simulink library "posemodel"  (R2019b)
settings: Solver=VariableStepAuto  StartTime=0.0  StopTime=10.0  RelTol=1e-3
libraries: posefilter x14, timecompensate x1

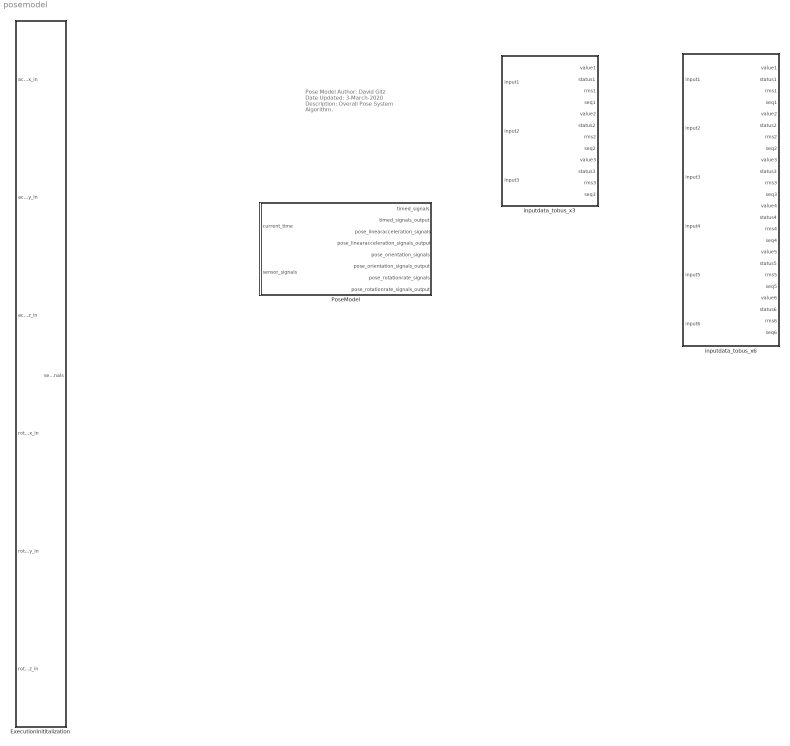
== system posemodel ==
  note: Pose Model
      | Author: David Gitz
      | Date Updated: 3-March-2020
      | Description:
      | Overall Pose System Algorithm.
  ExecutionInititalization : Subsystem
  PoseModel : Subsystem
  inputdata_tobus_x3 : MATLAB Function  TreatAsAtomicUnit=on
  inputdata_tobus_x6 : MATLAB Function  TreatAsAtomicUnit=on

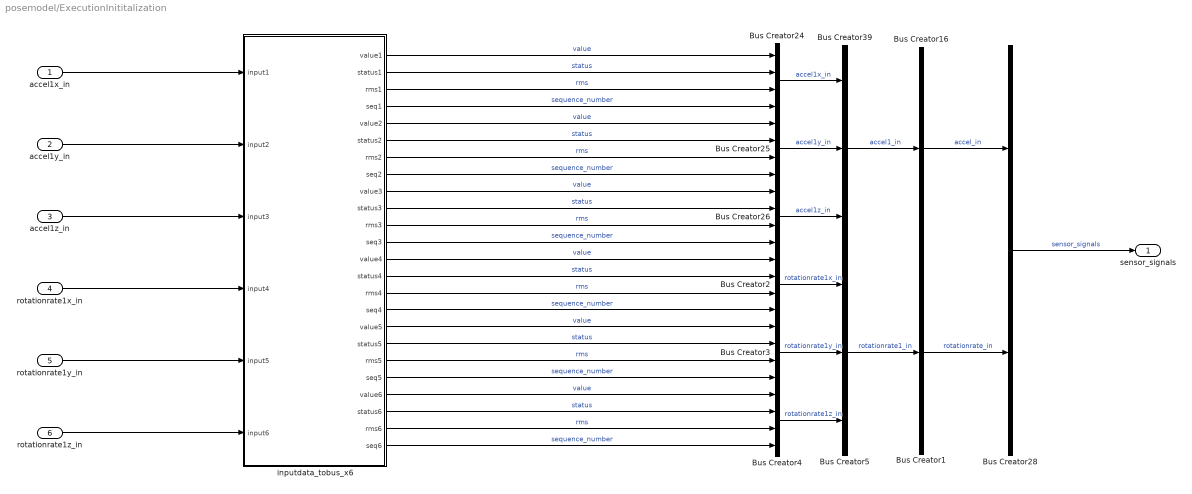
== system posemodel/ExecutionInititalization ==
  accel1x_in : Inport
  accel1y_in : Inport  Port=2
  accel1z_in : Inport  Port=3
  rotationrate1x_in : Inport  Port=4
  rotationrate1y_in : Inport  Port=5
  rotationrate1z_in : Inport  Port=6
  Bus Creator1 : BusCreator  Inputs=1
  Bus Creator16 : BusCreator  Inputs=1
  Bus Creator{2..4,24..26} (6 alike) : BusCreator  Inputs=4  OutDataTypeStr=Bus: InputSignalObject
  Bus Creator28 : BusCreator  Inputs=2
  Bus Creator39 : BusCreator  Inputs=3
  Bus Creator5 : BusCreator  Inputs=3
  inputdata_tobus_x6 : MATLAB Function  TreatAsAtomicUnit=on
  sensor_signals : Outport
  wires:
  inputdata_tobus_x6/20(seq5) -> Bus Creator3/4  "sequence_number"
  inputdata_tobus_x6/22(status6) -> Bus Creator4/2  "status"
  inputdata_tobus_x6/13(value4) -> Bus Creator2/1  "value"
  Bus Creator4/1 -> Bus Creator5/3  "rotationrate1z_in"
  Bus Creator1/1 -> Bus Creator28/2  "rotationrate_in"
  Bus Creator2/1 -> Bus Creator5/1  "rotationrate1x_in"
  inputdata_tobus_x6/23(rms6) -> Bus Creator4/3  "rms"
  inputdata_tobus_x6/14(status4) -> Bus Creator2/2  "status"
  inputdata_tobus_x6/21(value6) -> Bus Creator4/1  "value"
  inputdata_tobus_x6/19(rms5) -> Bus Creator3/3  "rms"
  inputdata_tobus_x6/17(value5) -> Bus Creator3/1  "value"
  Bus Creator5/1 -> Bus Creator1/1  "rotationrate1_in"
  inputdata_tobus_x6/16(seq4) -> Bus Creator2/4  "sequence_number"
  inputdata_tobus_x6/24(seq6) -> Bus Creator4/4  "sequence_number"
  inputdata_tobus_x6/15(rms4) -> Bus Creator2/3  "rms"
  inputdata_tobus_x6/18(status5) -> Bus Creator3/2  "status"
  Bus Creator3/1 -> Bus Creator5/2  "rotationrate1y_in"
  rotationrate1y_in/1 -> inputdata_tobus_x6/5(input5)
  rotationrate1z_in/1 -> inputdata_tobus_x6/6(input6)
  rotationrate1x_in/1 -> inputdata_tobus_x6/4(input4)
  inputdata_tobus_x6/3(rms1) -> Bus Creator24/3  "rms"
  inputdata_tobus_x6/5(value2) -> Bus Creator25/1  "value"
  inputdata_tobus_x6/2(status1) -> Bus Creator24/2  "status"
  inputdata_tobus_x6/4(seq1) -> Bus Creator24/4  "sequence_number"
  inputdata_tobus_x6/11(rms3) -> Bus Creator26/3  "rms"
  inputdata_tobus_x6/12(seq3) -> Bus Creator26/4  "sequence_number"
  Bus Creator39/1 -> Bus Creator16/1  "accel1_in"
  Bus Creator28/1 -> sensor_signals/1  "sensor_signals"
  accel1x_in/1 -> inputdata_tobus_x6/1(input1)
  inputdata_tobus_x6/6(status2) -> Bus Creator25/2  "status"
  accel1z_in/1 -> inputdata_tobus_x6/3(input3)
  Bus Creator24/1 -> Bus Creator39/1  "accel1x_in"
  Bus Creator16/1 -> Bus Creator28/1  "accel_in"
  Bus Creator25/1 -> Bus Creator39/2  "accel1y_in"
  inputdata_tobus_x6/9(value3) -> Bus Creator26/1  "value"
  inputdata_tobus_x6/7(rms2) -> Bus Creator25/3  "rms"
  inputdata_tobus_x6/8(seq2) -> Bus Creator25/4  "sequence_number"
  Bus Creator26/1 -> Bus Creator39/3  "accel1z_in"
  accel1y_in/1 -> inputdata_tobus_x6/2(input2)
  inputdata_tobus_x6/1(value1) -> Bus Creator24/1  "value"
  inputdata_tobus_x6/10(status3) -> Bus Creator26/2  "status"

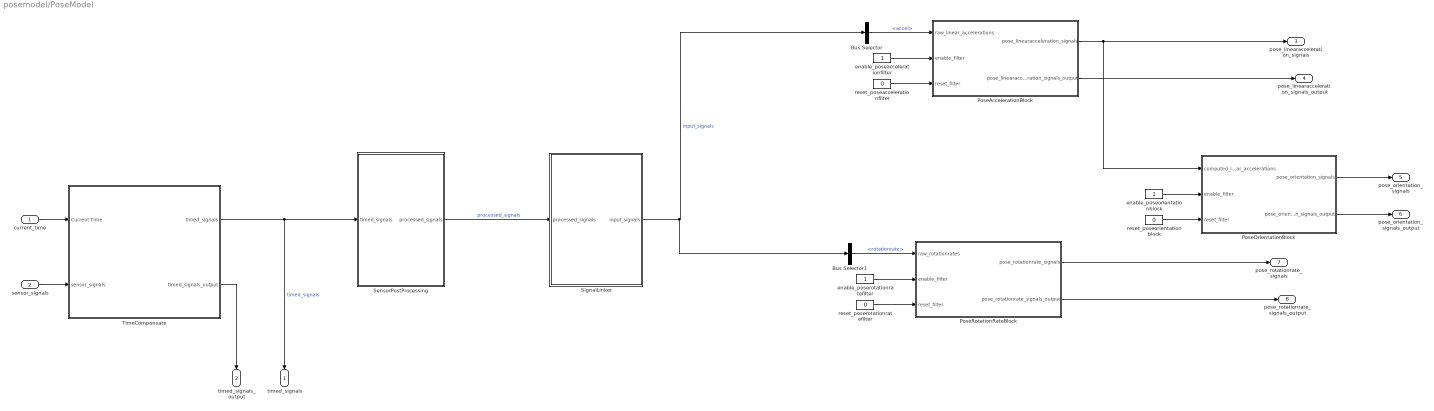
== system posemodel/PoseModel ==
  current_time : Inport
  sensor_signals : Inport  Port=2
  Bus Selector : BusSelector  OutputSignals=accel
  Bus Selector1 : BusSelector  OutputSignals=rotationrate
  PoseAccelerationBlock : Subsystem
  PoseOrientationBlock : Subsystem
  PoseRotationRateBlock : Subsystem
  SensorPostProcessing : Subsystem
  SignalLinker : Subsystem
  TimeCompensate : Subsystem  TreatAsAtomicUnit=on
  enable_poseaccelerationfilter : Constant
  enable_poseorientationblock : Constant
  enable_poserotationratefilter : Constant
  reset_poseaccelerationfilter : Constant  Value=0
  reset_poseorientationblock : Constant  Value=0
  reset_poserotationratefilter : Constant  Value=0
  timed_signals : Outport
  timed_signals_output : Outport  Port=2
  pose_linearacceleration_signals : Outport  Port=3
  pose_linearacceleration_signals_output : Outport  Port=4
  pose_orientation_signals : Outport  Port=5
  pose_orientation_signals_output : Outport  Port=6
  pose_rotationrate_signals : Outport  Port=7
  pose_rotationrate_signals_output : Outport  Port=8
  wires:
  PoseRotationRateBlock/1(pose_rotationrate_signals) -> pose_rotationrate_signals/1
  Bus Selector1/1 -> PoseRotationRateBlock/1(raw_rotationrates)  "<rotationrate>"
  enable_poserotationratefilter/1 -> PoseRotationRateBlock/2(enable_filter)
  reset_poserotationratefilter/1 -> PoseRotationRateBlock/3(reset_filter)
  PoseRotationRateBlock/2(pose_rotationrate_signals_output) -> pose_rotationrate_signals_output/1
  PoseAccelerationBlock/2(pose_linearacceleration_signals_output) -> pose_linearacceleration_signals_output/1
  TimeCompensate/2(timed_signals_output) -> timed_signals_output/1
  PoseOrientationBlock/2(pose_orientation_signals_output) -> pose_orientation_signals_output/1
  PoseOrientationBlock/1(pose_orientation_signals) -> pose_orientation_signals/1
  reset_poseorientationblock/1 -> PoseOrientationBlock/3(reset_filter)
  enable_poseorientationblock/1 -> PoseOrientationBlock/2(enable_filter)
  reset_poseaccelerationfilter/1 -> PoseAccelerationBlock/3(reset_filter)
  enable_poseaccelerationfilter/1 -> PoseAccelerationBlock/2(enable_filter)
  current_time/1 -> TimeCompensate/1(Current Time)
  Bus Selector/1 -> PoseAccelerationBlock/1(raw_linear_accelerations)  "<accel>"
  PoseAccelerationBlock/1(pose_linearacceleration_signals) -> pose_linearacceleration_signals/1, PoseOrientationBlock/1(computed_linear_accelerations)
  sensor_signals/1 -> TimeCompensate/2(sensor_signals)
  SensorPostProcessing/1(processed_signals) -> SignalLinker/1(processed_signals)  "processed_signals"
  SignalLinker/1(input_signals) -> Bus Selector/1, Bus Selector1/1  "input_signals"
  TimeCompensate/1(timed_signals) -> timed_signals/1, SensorPostProcessing/1(timed_signals)  "timed_signals"

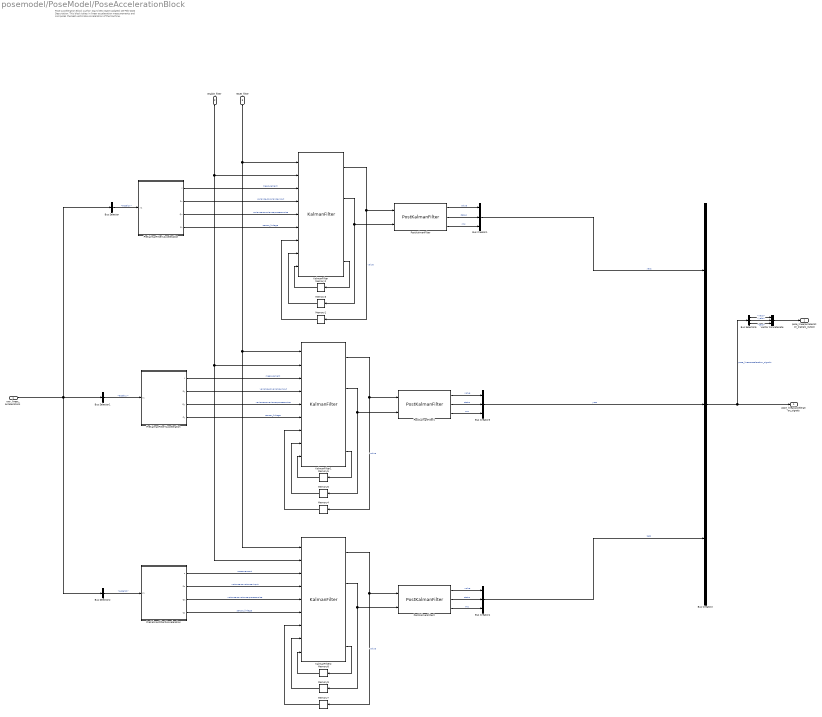
== system posemodel/PoseModel/PoseAccelerationBlock ==
  note: Pose Acceleration Block
      | Author: David Gitz
      | Date Updated: 28-Feb-2020
      | Description:
      | This block takes in linear acceleration measurements and computes the
      | best-estimate Acceleration of the Machine.
  raw_linear_accelerations : Inport
  enable_filter : Inport  Port=2
  reset_filter : Inport  Port=3
  Bus Creator1 : BusCreator  Inputs=3  OutDataTypeStr=Bus: OutputSignalObject  NonVirtualBus=on
  Bus Creator2 : BusCreator  Inputs=3
  Bus Creator3 : BusCreator  Inputs=3  OutDataTypeStr=Bus: OutputSignalObject  NonVirtualBus=on
  Bus Creator4 : BusCreator  Inputs=3  OutDataTypeStr=Bus: OutputSignalObject  NonVirtualBus=on
  Bus Selector : BusSelector  OutputSignals=accel1.accel1x
  Bus Selector1 : BusSelector  OutputSignals=accel1.accel1y
  Bus Selector2 : BusSelector  OutputSignals=accel1.accel1z
  Bus Selector6 : BusSelector  OutputSignals=xacc,yacc,zacc
  KalmanFilter : posefilter/KalmanFilter  SystemSampleTime=-1  Latency=0  AutoFrameSizeCalculation=off
  KalmanFilter1 : posefilter/KalmanFilter  SystemSampleTime=-1  Latency=0  AutoFrameSizeCalculation=off
  KalmanFilter2 : posefilter/KalmanFilter  SystemSampleTime=-1  Latency=0  AutoFrameSizeCalculation=off
  Memory{1..9} (9 alike) : Memory
  PostKalmanFilter : posefilter/PostKalmanFilter  SystemSampleTime=-1  Latency=0  AutoFrameSizeCalculation=off
  PostKalmanFilter1 : posefilter/PostKalmanFilter  SystemSampleTime=-1  Latency=0  AutoFrameSizeCalculation=off
  PostKalmanFilter2 : posefilter/PostKalmanFilter  SystemSampleTime=-1  Latency=0  AutoFrameSizeCalculation=off
  PreKalmanFilterXAcceleration : MATLAB Function  TreatAsAtomicUnit=on
  PreKalmanFilterYAcceleration : MATLAB Function  TreatAsAtomicUnit=on
  PreKalmanFilterZAcceleration : MATLAB Function  TreatAsAtomicUnit=on
  Vector Concatenate : Concatenate  NumInputs=3
  pose_linearacceleration_signals : Outport
  pose_linearacceleration_signals_output : Outport  Port=2
  wires:
  Vector Concatenate/1 -> pose_linearacceleration_signals_output/1
  Bus Selector6/3 -> Vector Concatenate/3  "<zacc>"
  Bus Selector6/2 -> Vector Concatenate/2  "<yacc>"
  Bus Selector6/1 -> Vector Concatenate/1  "<xacc>"
  Bus Creator2/1 -> pose_linearacceleration_signals/1, Bus Selector6/1  "pose_linearacceleration_signals"
  PostKalmanFilter2/3 -> Bus Creator4/3  "rms"
  Memory9/1 -> KalmanFilter2/8
  KalmanFilter2/1 -> PostKalmanFilter2/1, Memory7/1  "value"
  PreKalmanFilterZAcceleration/1(z) -> KalmanFilter2/3  "measurement"
  PostKalmanFilter2/1 -> Bus Creator4/1  "value"
  PreKalmanFilterZAcceleration/2(Rz) -> KalmanFilter2/4  "variance-covariance-input"
  PostKalmanFilter2/2 -> Bus Creator4/2  "status"
  raw_linear_accelerations/1 -> Bus Selector1/1, Bus Selector/1, Bus Selector2/1
  reset_filter/1 -> KalmanFilter/1, KalmanFilter1/1, KalmanFilter2/1
  Bus Selector2/1 -> PreKalmanFilterZAcceleration/1(x1)  "<accel1z>"
  KalmanFilter2/4 -> Memory8/1
  KalmanFilter2/2 -> Memory9/1, PostKalmanFilter2/2
  Bus Creator4/1 -> Bus Creator2/3  "zacc"
  enable_filter/1 -> KalmanFilter/2, KalmanFilter1/2, KalmanFilter2/2
  PreKalmanFilterZAcceleration/3(Qz) -> KalmanFilter2/5  "variance-covariance-processnoise"
  Memory8/1 -> KalmanFilter2/9
  Memory7/1 -> KalmanFilter2/7
  PreKalmanFilterZAcceleration/4(Cz) -> KalmanFilter2/6  "sensor_linkage"
  Bus Creator3/1 -> Bus Creator2/2  "yacc"
  PreKalmanFilterYAcceleration/1(y) -> KalmanFilter1/3  "measurement"
  PostKalmanFilter1/3 -> Bus Creator3/3  "rms"
  Memory6/1 -> KalmanFilter1/8
  PostKalmanFilter1/2 -> Bus Creator3/2  "status"
  PostKalmanFilter1/1 -> Bus Creator3/1  "value"
  PreKalmanFilterYAcceleration/2(Ry) -> KalmanFilter1/4  "variance-covariance-input"
  Memory4/1 -> KalmanFilter1/7
  PreKalmanFilterYAcceleration/3(Qy) -> KalmanFilter1/5  "variance-covariance-processnoise"
  PreKalmanFilterYAcceleration/4(Cy) -> KalmanFilter1/6  "sensor_linkage"
  Bus Selector1/1 -> PreKalmanFilterYAcceleration/1(x1)  "<accel1y>"
  KalmanFilter1/1 -> PostKalmanFilter1/1, Memory4/1  "value"
  KalmanFilter1/2 -> Memory6/1, PostKalmanFilter1/2
  KalmanFilter1/4 -> Memory5/1
  Memory5/1 -> KalmanFilter1/9
  PreKalmanFilterXAcceleration/3(Qx) -> KalmanFilter/5  "variance-covariance-processnoise"
  PreKalmanFilterXAcceleration/1(x) -> KalmanFilter/3  "measurement"
  PreKalmanFilterXAcceleration/4(Cx) -> KalmanFilter/6  "sensor_linkage"
  KalmanFilter/2 -> Memory3/1, PostKalmanFilter/2
  Memory3/1 -> KalmanFilter/8
  Bus Selector/1 -> PreKalmanFilterXAcceleration/1(x1)  "<accel1x>"
  PostKalmanFilter/2 -> Bus Creator1/2  "status"
  PostKalmanFilter/1 -> Bus Creator1/1  "value"
  PostKalmanFilter/3 -> Bus Creator1/3  "rms"
  Memory2/1 -> KalmanFilter/9
  Memory1/1 -> KalmanFilter/7
  PreKalmanFilterXAcceleration/2(Rx) -> KalmanFilter/4  "variance-covariance-input"
  KalmanFilter/4 -> Memory2/1
  Bus Creator1/1 -> Bus Creator2/1  "xacc"
  KalmanFilter/1 -> PostKalmanFilter/1, Memory1/1  "value"

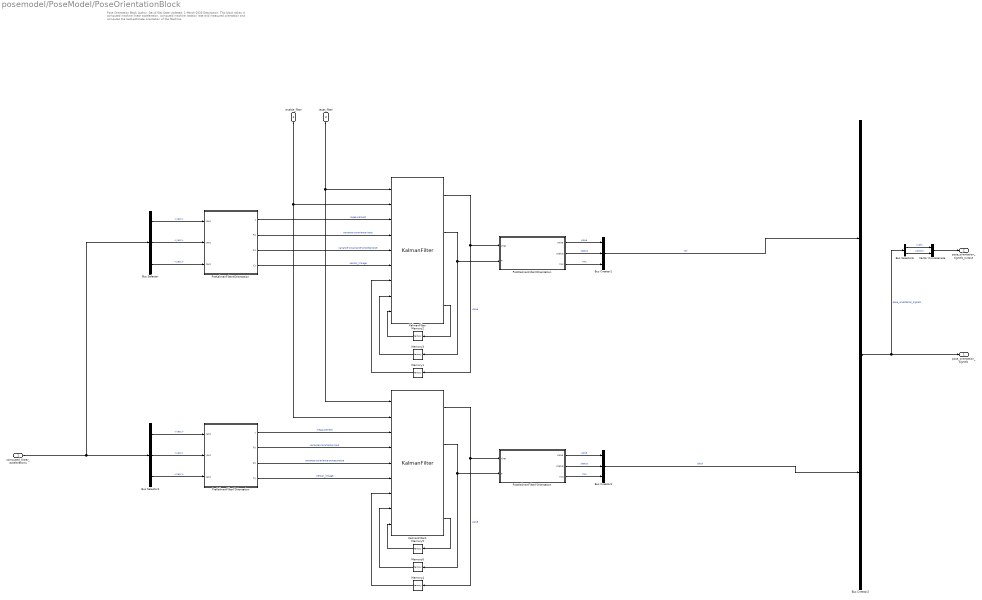
== system posemodel/PoseModel/PoseOrientationBlock ==
  note: Pose Orientation Block
      | Author: David Gitz
      | Date Updated: 1-March-2020
      | Description:
      | This block takes in computed machine linear acceleration, computed machine rotation rate and measured orientation and computes the
      | best-estimate orientation of the Machine.
  computed_linear_accelerations : Inport
  enable_filter : Inport  Port=2
  reset_filter : Inport  Port=3
  Bus Creator1 : BusCreator  Inputs=3  OutDataTypeStr=Bus: OutputSignalObject  NonVirtualBus=on
  Bus Creator2 : BusCreator  Inputs=2
  Bus Creator3 : BusCreator  Inputs=3  OutDataTypeStr=Bus: OutputSignalObject  NonVirtualBus=on
  Bus Selector : BusSelector  OutputSignals=xacc,yacc,zacc
  Bus Selector1 : BusSelector  OutputSignals=xacc,yacc,zacc
  Bus Selector6 : BusSelector  OutputSignals=roll,pitch
  KalmanFilter : posefilter/KalmanFilter  SystemSampleTime=-1  Latency=0  AutoFrameSizeCalculation=off
  KalmanFilter1 : posefilter/KalmanFilter  SystemSampleTime=-1  Latency=0  AutoFrameSizeCalculation=off
  Memory{1..6} (6 alike) : Memory
  PostKalmanFilterXOrientation : MATLAB Function  TreatAsAtomicUnit=on
  PostKalmanFilterYOrientation : MATLAB Function  TreatAsAtomicUnit=on
  PreKalmanFilterXOrientation : MATLAB Function  TreatAsAtomicUnit=on
  PreKalmanFilterYOrientation : MATLAB Function  TreatAsAtomicUnit=on
  Vector Concatenate : Concatenate
  pose_orientation_signals : Outport
  pose_orientation_signals_output : Outport  Port=2
  wires:
  Bus Selector6/2 -> Vector Concatenate/2  "<pitch>"
  Bus Selector6/1 -> Vector Concatenate/1  "<roll>"
  Vector Concatenate/1 -> pose_orientation_signals_output/1
  Bus Creator2/1 -> pose_orientation_signals/1, Bus Selector6/1  "pose_orientation_signals"
  Bus Creator3/1 -> Bus Creator2/2  "pitch"
  Memory6/1 -> KalmanFilter1/8
  KalmanFilter1/2 -> PostKalmanFilterYOrientation/2(P), Memory6/1
  Bus Selector1/3 -> PreKalmanFilterYOrientation/3(zacc)  "<zacc>"
  Bus Selector1/2 -> PreKalmanFilterYOrientation/2(yacc)  "<yacc>"
  Memory4/1 -> KalmanFilter1/7
  PostKalmanFilterYOrientation/3(rms) -> Bus Creator3/3  "rms"
  PreKalmanFilterYOrientation/1(y) -> KalmanFilter1/3  "measurement"
  PreKalmanFilterYOrientation/3(Qy) -> KalmanFilter1/5  "variance-covariance-processnoise"
  PreKalmanFilterYOrientation/2(Ry) -> KalmanFilter1/4  "variance-covariance-input"
  enable_filter/1 -> KalmanFilter/2, KalmanFilter1/2
  Bus Selector1/1 -> PreKalmanFilterYOrientation/1(xacc)  "<xacc>"
  PreKalmanFilterYOrientation/4(Cy) -> KalmanFilter1/6  "sensor_linkage"
  PostKalmanFilterYOrientation/1(value) -> Bus Creator3/1  "value"
  PostKalmanFilterYOrientation/2(status) -> Bus Creator3/2  "status"
  KalmanFilter1/4 -> Memory5/1
  computed_linear_accelerations/1 -> Bus Selector/1, Bus Selector1/1
  reset_filter/1 -> KalmanFilter/1, KalmanFilter1/1
  Memory5/1 -> KalmanFilter1/9
  KalmanFilter1/1 -> Memory4/1, PostKalmanFilterYOrientation/1(xhat)  "value"
  Bus Selector/3 -> PreKalmanFilterXOrientation/3(zacc)  "<zacc>"
  Bus Selector/2 -> PreKalmanFilterXOrientation/2(yacc)  "<yacc>"
  Bus Selector/1 -> PreKalmanFilterXOrientation/1(xacc)  "<xacc>"
  Memory3/1 -> KalmanFilter/8
  KalmanFilter/1 -> Memory1/1, PostKalmanFilterXOrientation/1(xhat)  "value"
  Bus Creator1/1 -> Bus Creator2/1  "roll"
  PostKalmanFilterXOrientation/1(value) -> Bus Creator1/1  "value"
  PostKalmanFilterXOrientation/3(rms) -> Bus Creator1/3  "rms"
  KalmanFilter/4 -> Memory2/1
  PreKalmanFilterXOrientation/4(Cx) -> KalmanFilter/6  "sensor_linkage"
  PostKalmanFilterXOrientation/2(status) -> Bus Creator1/2  "status"
  PreKalmanFilterXOrientation/1(x) -> KalmanFilter/3  "measurement"
  Memory1/1 -> KalmanFilter/7
  PreKalmanFilterXOrientation/3(Qx) -> KalmanFilter/5  "variance-covariance-processnoise"
  PreKalmanFilterXOrientation/2(Rx) -> KalmanFilter/4  "variance-covariance-input"
  KalmanFilter/2 -> PostKalmanFilterXOrientation/2(P), Memory3/1
  Memory2/1 -> KalmanFilter/9

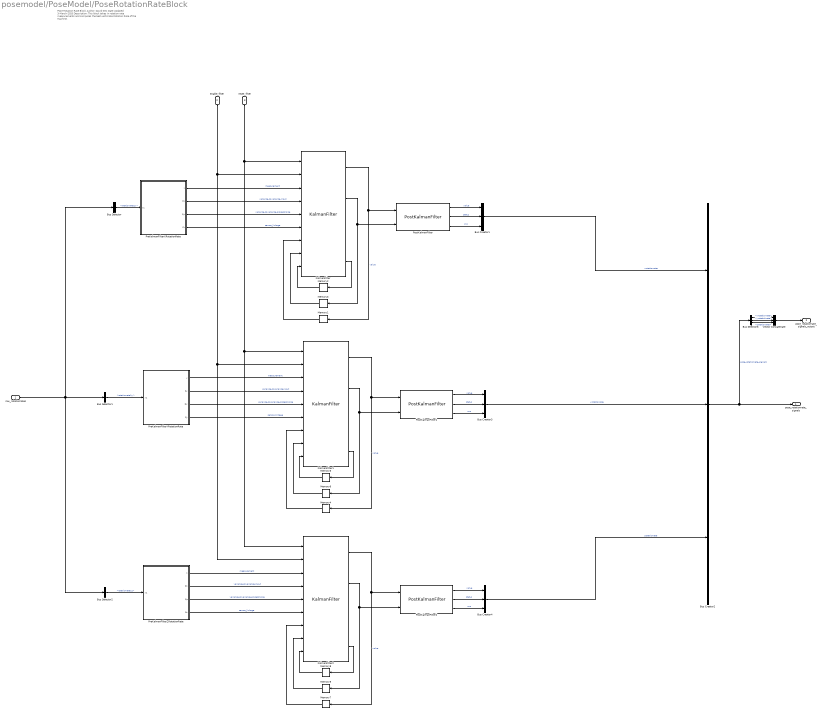
== system posemodel/PoseModel/PoseRotationRateBlock ==
  note: Pose Rotation Rate Block
      | Author: David Gitz
      | Date Updated: 3-March-2020
      | Description:
      | This block takes in rotation rate measurements and computes the
      | best-estimate Rotation Rate of the Machine.
  raw_rotationrates : Inport
  enable_filter : Inport  Port=2
  reset_filter : Inport  Port=3
  Bus Creator1 : BusCreator  Inputs=3  OutDataTypeStr=Bus: OutputSignalObject  NonVirtualBus=on
  Bus Creator2 : BusCreator  Inputs=3
  Bus Creator3 : BusCreator  Inputs=3  OutDataTypeStr=Bus: OutputSignalObject  NonVirtualBus=on
  Bus Creator4 : BusCreator  Inputs=3  OutDataTypeStr=Bus: OutputSignalObject  NonVirtualBus=on
  Bus Selector : BusSelector  OutputSignals=rotationrate1.rotationrate1x
  Bus Selector1 : BusSelector  OutputSignals=rotationrate1.rotationrate1y
  Bus Selector2 : BusSelector  OutputSignals=rotationrate1.rotationrate1z
  Bus Selector6 : BusSelector  OutputSignals=xrotationrate,yrotationrate,zrotationrate
  KalmanFilter : posefilter/KalmanFilter  SystemSampleTime=-1  Latency=0  AutoFrameSizeCalculation=off
  KalmanFilter1 : posefilter/KalmanFilter  SystemSampleTime=-1  Latency=0  AutoFrameSizeCalculation=off
  KalmanFilter2 : posefilter/KalmanFilter  SystemSampleTime=-1  Latency=0  AutoFrameSizeCalculation=off
  Memory{1..9} (9 alike) : Memory
  PostKalmanFilter : posefilter/PostKalmanFilter  SystemSampleTime=-1  Latency=0  AutoFrameSizeCalculation=off
  PostKalmanFilter1 : posefilter/PostKalmanFilter  SystemSampleTime=-1  Latency=0  AutoFrameSizeCalculation=off
  PostKalmanFilter2 : posefilter/PostKalmanFilter  SystemSampleTime=-1  Latency=0  AutoFrameSizeCalculation=off
  PreKalmanFilterXRotationRate : MATLAB Function  TreatAsAtomicUnit=on
  PreKalmanFilterYRotationRate : MATLAB Function  TreatAsAtomicUnit=on
  PreKalmanFilterZRotationRate : MATLAB Function  TreatAsAtomicUnit=on
  Vector Concatenate : Concatenate  NumInputs=3
  pose_rotationrate_signals : Outport
  pose_rotationrate_signals_output : Outport  Port=2
  wires:
  KalmanFilter/1 -> Memory1/1, PostKalmanFilter/1  "value"
  Bus Creator1/1 -> Bus Creator2/1  "xrotationrate"
  KalmanFilter/4 -> Memory2/1
  PreKalmanFilterXRotationRate/2(Rx) -> KalmanFilter/4  "variance-covariance-input"
  Memory1/1 -> KalmanFilter/7
  Memory2/1 -> KalmanFilter/9
  PostKalmanFilter/3 -> Bus Creator1/3  "rms"
  PostKalmanFilter/1 -> Bus Creator1/1  "value"
  PostKalmanFilter/2 -> Bus Creator1/2  "status"
  Bus Selector/1 -> PreKalmanFilterXRotationRate/1(x1)  "<rotationrate1x>"
  Memory3/1 -> KalmanFilter/8
  KalmanFilter/2 -> PostKalmanFilter/2, Memory3/1
  PreKalmanFilterXRotationRate/4(Cx) -> KalmanFilter/6  "sensor_linkage"
  PreKalmanFilterXRotationRate/1(x) -> KalmanFilter/3  "measurement"
  PreKalmanFilterXRotationRate/3(Qx) -> KalmanFilter/5  "variance-covariance-processnoise"
  Memory5/1 -> KalmanFilter1/9
  KalmanFilter1/4 -> Memory5/1
  KalmanFilter1/2 -> PostKalmanFilter1/2, Memory6/1
  KalmanFilter1/1 -> Memory4/1, PostKalmanFilter1/1  "value"
  Bus Selector1/1 -> PreKalmanFilterYRotationRate/1(x1)  "<rotationrate1y>"
  PreKalmanFilterYRotationRate/4(Cy) -> KalmanFilter1/6  "sensor_linkage"
  PreKalmanFilterYRotationRate/3(Qy) -> KalmanFilter1/5  "variance-covariance-processnoise"
  Memory4/1 -> KalmanFilter1/7
  PreKalmanFilterYRotationRate/2(Ry) -> KalmanFilter1/4  "variance-covariance-input"
  PostKalmanFilter1/1 -> Bus Creator3/1  "value"
  PostKalmanFilter1/2 -> Bus Creator3/2  "status"
  Memory6/1 -> KalmanFilter1/8
  PostKalmanFilter1/3 -> Bus Creator3/3  "rms"
  PreKalmanFilterYRotationRate/1(y) -> KalmanFilter1/3  "measurement"
  Bus Creator3/1 -> Bus Creator2/2  "yrotationrate"
  PreKalmanFilterZRotationRate/4(Cz) -> KalmanFilter2/6  "sensor_linkage"
  Memory7/1 -> KalmanFilter2/7
  Memory8/1 -> KalmanFilter2/9
  PreKalmanFilterZRotationRate/3(Qz) -> KalmanFilter2/5  "variance-covariance-processnoise"
  enable_filter/1 -> KalmanFilter2/2, KalmanFilter1/2, KalmanFilter/2
  Bus Creator4/1 -> Bus Creator2/3  "zrotationrate"
  KalmanFilter2/2 -> PostKalmanFilter2/2, Memory9/1
  KalmanFilter2/4 -> Memory8/1
  Bus Selector2/1 -> PreKalmanFilterZRotationRate/1(x1)  "<rotationrate1z>"
  reset_filter/1 -> KalmanFilter2/1, KalmanFilter1/1, KalmanFilter/1
  raw_rotationrates/1 -> Bus Selector2/1, Bus Selector/1, Bus Selector1/1
  PostKalmanFilter2/2 -> Bus Creator4/2  "status"
  PreKalmanFilterZRotationRate/2(Rz) -> KalmanFilter2/4  "variance-covariance-input"
  PostKalmanFilter2/1 -> Bus Creator4/1  "value"
  PreKalmanFilterZRotationRate/1(z) -> KalmanFilter2/3  "measurement"
  KalmanFilter2/1 -> Memory7/1, PostKalmanFilter2/1  "value"
  Memory9/1 -> KalmanFilter2/8
  PostKalmanFilter2/3 -> Bus Creator4/3  "rms"
  Bus Creator2/1 -> Bus Selector6/1, pose_rotationrate_signals/1  "pose_rotationrate_signals"
  Bus Selector6/1 -> Vector Concatenate/1  "<xrotationrate>"
  Bus Selector6/2 -> Vector Concatenate/2  "<yrotationrate>"
  Bus Selector6/3 -> Vector Concatenate/3  "<zrotationrate>"
  Vector Concatenate/1 -> pose_rotationrate_signals_output/1

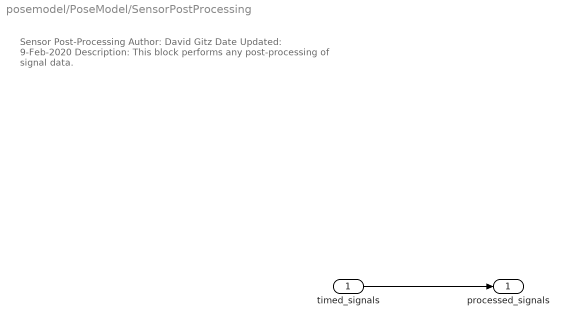
== system posemodel/PoseModel/SensorPostProcessing ==
  note: Sensor Post-Processing
      | Author: David Gitz
      | Date Updated: 9-Feb-2020
      | Description:
      | This block performs any post-processing of signal data.
  timed_signals : Inport
  processed_signals : Outport
  wires:
  timed_signals/1 -> processed_signals/1

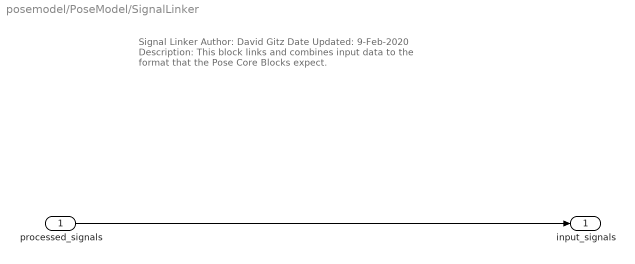
== system posemodel/PoseModel/SignalLinker ==
  note: Signal Linker
      | Author: David Gitz
      | Date Updated: 9-Feb-2020
      | Description:
      | This block links and combines input data to the format that
      | the Pose Core Blocks expect.
  processed_signals : Inport
  input_signals : Outport
  wires:
  processed_signals/1 -> input_signals/1

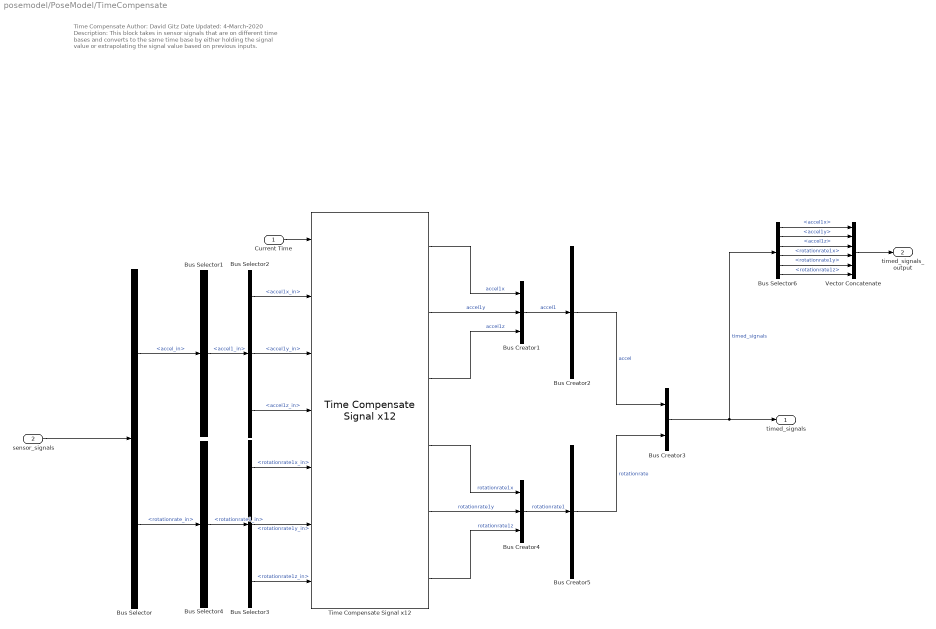
== system posemodel/PoseModel/TimeCompensate ==
  note: Time Compensate
      | Author: David Gitz
      | Date Updated: 4-March-2020
      | Description:
      | This block takes in sensor signals that are on different time bases
      | and converts to the same time base by either holding the signal value
      | or extrapolating the signal value based on previous inputs.
  Current Time : Inport
  sensor_signals : Inport  Port=2
  Bus Creator1 : BusCreator  Inputs=3
  Bus Creator2 : BusCreator  Inputs=1
  Bus Creator3 : BusCreator  Inputs=2
  Bus Creator4 : BusCreator  Inputs=3
  Bus Creator5 : BusCreator  Inputs=1
  Bus Selector : BusSelector  OutputSignals=accel_in,rotationrate_in
  Bus Selector1 : BusSelector  OutputSignals=accel1_in
  Bus Selector2 : BusSelector  OutputSignals=accel1x_in,accel1y_in,accel1z_in
  Bus Selector3 : BusSelector  OutputSignals=rotationrate1x_in,rotationrate1y_in,rotationrate1z_in
  Bus Selector4 : BusSelector  OutputSignals=rotationrate1_in
  Bus Selector6 : BusSelector  OutputSignals=accel.accel1.accel1x,accel.accel1.accel1y,accel.accel1.accel1z,rotationrate.rotationrate1.rotationrate1x,rotationrate.rotationrate1.rotationrate1y,rotationrate.rotationrate1.rotationrate1z
  Time Compensate Signal x12 : timecompensate/Time Compensate Signal x12  SystemSampleTime=-1  Latency=0  AutoFrameSizeCalculation=off
  Vector Concatenate : Concatenate  NumInputs=6
  timed_signals : Outport
  timed_signals_output : Outport  Port=2
  wires:
  Bus Selector6/6 -> Vector Concatenate/6  "<rotationrate1z>"
  Bus Selector6/5 -> Vector Concatenate/5  "<rotationrate1y>"
  Bus Selector6/4 -> Vector Concatenate/4  "<rotationrate1x>"
  Bus Selector6/3 -> Vector Concatenate/3  "<accel1z>"
  Bus Selector6/2 -> Vector Concatenate/2  "<accel1y>"
  Bus Selector6/1 -> Vector Concatenate/1  "<accel1x>"
  Vector Concatenate/1 -> timed_signals_output/1
  Bus Creator3/1 -> timed_signals/1, Bus Selector6/1  "timed_signals"
  Time Compensate Signal x12/4 -> Bus Creator4/1  "rotationrate1x"
  Time Compensate Signal x12/6 -> Bus Creator4/3  "rotationrate1z"
  Bus Creator4/1 -> Bus Creator5/1  "rotationrate1"
  Bus Creator5/1 -> Bus Creator3/2  "rotationrate"
  Time Compensate Signal x12/5 -> Bus Creator4/2  "rotationrate1y"
  Bus Selector4/1 -> Bus Selector3/1  "<rotationrate1_in>"
  Bus Selector/2 -> Bus Selector4/1  "<rotationrate_in>"
  Bus Selector3/3 -> Time Compensate Signal x12/7  "<rotationrate1z_in>"
  Bus Selector3/2 -> Time Compensate Signal x12/6  "<rotationrate1y_in>"
  Bus Selector3/1 -> Time Compensate Signal x12/5  "<rotationrate1x_in>"
  Current Time/1 -> Time Compensate Signal x12/1
  sensor_signals/1 -> Bus Selector/1
  Bus Selector/1 -> Bus Selector1/1  "<accel_in>"
  Bus Selector1/1 -> Bus Selector2/1  "<accel1_in>"
  Time Compensate Signal x12/1 -> Bus Creator1/1  "accel1x"
  Bus Selector2/1 -> Time Compensate Signal x12/2  "<accel1x_in>"
  Bus Selector2/2 -> Time Compensate Signal x12/3  "<accel1y_in>"
  Bus Selector2/3 -> Time Compensate Signal x12/4  "<accel1z_in>"
  Time Compensate Signal x12/2 -> Bus Creator1/2  "accel1y"
  Time Compensate Signal x12/3 -> Bus Creator1/3  "accel1z"
  Bus Creator1/1 -> Bus Creator2/1  "accel1"
  Bus Creator2/1 -> Bus Creator3/1  "accel"

== matlab function posemodel/inputdata_tobus_x3 ==
function [value1,status1,rms1,seq1, ... 
            value2,status2,rms2,seq2, ... 
            value3,status3,rms3,seq3] ...
              = inputdata_tobus_x3( ...
                input1,input2,input3)
VALUE_INDEX = 1;
STATUS_INDEX = 2;
RMS_INDEX = 3;
SEQUENCENUMBER_INDEX = 4;

value1 = input1(VALUE_INDEX);
status1 = input1(STATUS_INDEX);
rms1 = input1(RMS_INDEX);
seq1 = input1(SEQUENCENUMBER_INDEX);

value2 = input2(VALUE_INDEX);
status2 = input2(STATUS_INDEX);
rms2 = input2(RMS_INDEX);
seq2 = input2(SEQUENCENUMBER_INDEX);

value3 = input3(VALUE_INDEX);
status3 = input3(STATUS_INDEX);
rms3 = input3(RMS_INDEX);
seq3 = input3(SEQUENCENUMBER_INDEX);
end

== matlab function posemodel/ExecutionInititalization/inputdata_tobus_x6 ==
function [value1,status1,rms1,seq1, ... 
            value2,status2,rms2,seq2, ... 
            value3,status3,rms3,seq3, ...
            value4,status4,rms4,seq4, ...
            value5,status5,rms5,seq5, ...
            value6,status6,rms6,seq6] ...
              = inputdata_tobus_x6( ...
                input1,input2,input3,input4,input5,input6)
VALUE_INDEX = 1;
STATUS_INDEX = 2;
RMS_INDEX = 3;
SEQUENCENUMBER_INDEX = 4;

value1 = input1(VALUE_INDEX);
status1 = input1(STATUS_INDEX);
rms1 = input1(RMS_INDEX);
seq1 = input1(SEQUENCENUMBER_INDEX);

value2 = input2(VALUE_INDEX);
status2 = input2(STATUS_INDEX);
rms2 = input2(RMS_INDEX);
seq2 = input2(SEQUENCENUMBER_INDEX);

value3 = input3(VALUE_INDEX);
status3 = input3(STATUS_INDEX);
rms3 = input3(RMS_INDEX);
seq3 = input3(SEQUENCENUMBER_INDEX);

value4 = input4(VALUE_INDEX);
status4 = input4(STATUS_INDEX);
rms4 = input4(RMS_INDEX);
seq4 = input4(SEQUENCENUMBER_INDEX);

value5 = input5(VALUE_INDEX);
status5 = input5(STATUS_INDEX);
rms5 = input5(RMS_INDEX);
seq5 = input5(SEQUENCENUMBER_INDEX);

value6 = input6(VALUE_INDEX);
status6 = input6(STATUS_INDEX);
rms6 = input6(RMS_INDEX);
seq6 = input6(SEQUENCENUMBER_INDEX);
end

== matlab function posemodel/PoseModel/PoseAccelerationBlock/PreKalmanFilterXAcceleration ==
function [x,Rx,Qx,Cx] = PreKalmanFilterXAcceleration(x1)
x = x1.value;
Rx = KalmanFilterAccelerationConfig.XAcc_R;
Qx = KalmanFilterAccelerationConfig.XAcc_Q;
Cx = KalmanFilterAccelerationConfig.XAcc_C;

== matlab function posemodel/PoseModel/PoseAccelerationBlock/PreKalmanFilterYAcceleration ==
function [y,Ry,Qy,Cy] = PreKalmanFilterYAcceleration(x1)
y = x1.value;
Ry = KalmanFilterAccelerationConfig.YAcc_R;
Qy = KalmanFilterAccelerationConfig.YAcc_Q;
Cy = KalmanFilterAccelerationConfig.YAcc_C;

== matlab function posemodel/PoseModel/PoseAccelerationBlock/PreKalmanFilterZAcceleration ==
function [z,Rz,Qz,Cz] = PreKalmanFilterZAcceleration(x1)
z = x1.value;
Rz = KalmanFilterAccelerationConfig.ZAcc_R;
Qz = KalmanFilterAccelerationConfig.ZAcc_Q;
Cz = KalmanFilterAccelerationConfig.ZAcc_C;

== matlab function posemodel/PoseModel/PoseOrientationBlock/PreKalmanFilterXOrientation ==
function [x,Rx,Qx,Cx] = PreKalmanFilterXOrientation(xacc,yacc,zacc)
% Compute Acceleration-Based Roll
mu = 0.01;
roll_acc = atan2(yacc.value,(sign(zacc.value)*((zacc.value*zacc.value)+mu*(xacc.value*xacc.value))^0.5));
Rx_acc = KalmanFilterOrientationConfig.XOrientation_R;
Qx_acc = KalmanFilterOrientationConfig.XOrientation_Q;
Cx_acc = KalmanFilterOrientationConfig.XOrientation_C;

x = [roll_acc];
Rx = [Rx_acc];
Qx = [Qx_acc];
Cx = [Cx_acc];

== matlab function posemodel/PoseModel/PoseOrientationBlock/PostKalmanFilterXOrientation ==
function [value,status, rms]  = PostKalmanFilterXOrientation(xhat,P)

value =xhat*180.0/pi;
status = uint8(SignalState.SIGNALSTATE_UPDATED_);
rms = P;

== matlab function posemodel/PoseModel/PoseOrientationBlock/PostKalmanFilterYOrientation ==
function [value,status, rms]  = PostKalmanFilterYOrientation(xhat,P)

value =xhat*180.0/pi;
status = uint8(SignalState.SIGNALSTATE_UPDATED_);
rms = P;

== matlab function posemodel/PoseModel/PoseOrientationBlock/PreKalmanFilterYOrientation ==
function [y,Ry,Qy,Cy] = PreKalmanFilterYOrientation(xacc,yacc,zacc)
% Compute Acceleration-Based Pitch
pitch_acc = atan2(-xacc.value,(((yacc.value*yacc.value) + (zacc.value*zacc.value))^0.5));
Ry_acc = KalmanFilterOrientationConfig.YOrientation_R;
Qy_acc = KalmanFilterOrientationConfig.YOrientation_Q;
Cy_acc = KalmanFilterOrientationConfig.YOrientation_C;

y = [pitch_acc];
Ry = [Ry_acc];
Qy = [Qy_acc];
Cy = [Cy_acc];

== matlab function posemodel/inputdata_tobus_x6 ==
function [value1,status1,rms1,seq1, ... 
            value2,status2,rms2,seq2, ... 
            value3,status3,rms3,seq3, ...
            value4,status4,rms4,seq4, ...
            value5,status5,rms5,seq5, ...
            value6,status6,rms6,seq6] ...
              = inputdata_tobus_x6( ...
                input1,input2,input3,input4,input5,input6)
VALUE_INDEX = 1;
STATUS_INDEX = 2;
RMS_INDEX = 3;
SEQUENCENUMBER_INDEX = 4;

value1 = input1(VALUE_INDEX);
status1 = input1(STATUS_INDEX);
rms1 = input1(RMS_INDEX);
seq1 = input1(SEQUENCENUMBER_INDEX);

value2 = input2(VALUE_INDEX);
status2 = input2(STATUS_INDEX);
rms2 = input2(RMS_INDEX);
seq2 = input2(SEQUENCENUMBER_INDEX);

value3 = input3(VALUE_INDEX);
status3 = input3(STATUS_INDEX);
rms3 = input3(RMS_INDEX);
seq3 = input3(SEQUENCENUMBER_INDEX);

value4 = input4(VALUE_INDEX);
status4 = input4(STATUS_INDEX);
rms4 = input4(RMS_INDEX);
seq4 = input4(SEQUENCENUMBER_INDEX);

value5 = input5(VALUE_INDEX);
status5 = input5(STATUS_INDEX);
rms5 = input5(RMS_INDEX);
seq5 = input5(SEQUENCENUMBER_INDEX);

value6 = input6(VALUE_INDEX);
status6 = input6(STATUS_INDEX);
rms6 = input6(RMS_INDEX);
seq6 = input6(SEQUENCENUMBER_INDEX);
end

== matlab function posemodel/PoseModel/PoseRotationRateBlock/PreKalmanFilterXRotationRate ==
function [x,Rx,Qx,Cx] = PreKalmanFilterXRotationRate(x1)
x = x1.value;
Rx = KalmanFilterRotationRateConfig.XRotationRate_R;
Qx = KalmanFilterRotationRateConfig.XRotationRate_Q;
Cx = KalmanFilterRotationRateConfig.XRotationRate_C;

== matlab function posemodel/PoseModel/PoseRotationRateBlock/PreKalmanFilterYRotationRate ==
function [y,Ry,Qy,Cy] = PreKalmanFilterYRotationRate(x1)
y = x1.value;
Ry = KalmanFilterRotationRateConfig.YRotationRate_R;
Qy = KalmanFilterRotationRateConfig.YRotationRate_Q;
Cy = KalmanFilterRotationRateConfig.YRotationRate_C;

== matlab function posemodel/PoseModel/PoseRotationRateBlock/PreKalmanFilterZRotationRate ==
function [z,Rz,Qz,Cz] = PreKalmanFilterZRotationRate(x1)
z = x1.value;
Rz = KalmanFilterRotationRateConfig.ZRotationRate_R;
Qz = KalmanFilterRotationRateConfig.ZRotationRate_Q;
Cz = KalmanFilterRotationRateConfig.ZRotationRate_C;
